simulink model "etc_r2v_subs"  (Simulink 7.0)
settings: Solver=FixedStepDiscrete  StartTime=0.0  StopTime=10.0  RelTol=1e-3
PreLoadFcn:
  | t = linspace(0,10,101)';
  | u = linspace(0,pi/2,101)';
settings Model: Creator=jrivitus  LastModifiedBy=jrivitus
settings DataIOCC: LoadExternalInput=on
settings OptimizationCC: InitFltsAndDblsToZero=off

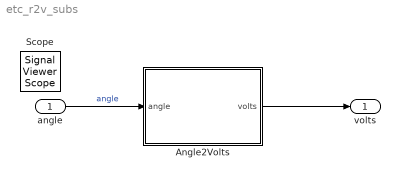
== system etc_r2v_subs ==
  "angle " : Inport  OutDataType=sfix(16)  OutScaling=2^0
  Angle2Volts : Subsystem
  volts : Outport  OutDataType=sfix(16)  OutScaling=2^0
  Scope : SignalViewerScope  IOType=viewer  RefreshTime=0.035000
      settings: TimeRange=10  YMin=0  YMax=100
  wires:
  Angle2Volts/1(volts) -> volts/1
  "angle "/1 -> Angle2Volts/1("angle ")  "angle"

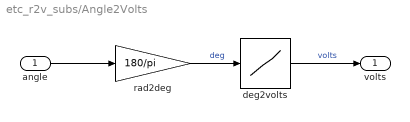
== system etc_r2v_subs/Angle2Volts ==
  "angle " : Inport  OutDataType=sfix(16)  OutScaling=2^0
  deg2volts : Lookup  InputValues=[0 90]  Table=[0.5 4.5]  OutDataType=sfix(16)  OutScaling=2^0
  rad2deg : Gain  Gain=180/pi  ParameterDataType=sfix(16)  ParameterScaling=2^0  OutDataType=sfix(16)  OutScaling=2^0  SaturateOnIntegerOverflow=on
  volts : Outport  OutDataType=sfix(16)  OutScaling=2^0
  wires:
  "angle "/1 -> rad2deg/1
  deg2volts/1 -> volts/1  "volts"
  rad2deg/1 -> deg2volts/1  "deg"
